simulink library "SignalSourceBlockLibrary"  (R2022b)
settings: Solver=VariableStepAuto  StartTime=0.0  StopTime=10.0  RelTol=1e-3
settings Model: Creator=isaacito  LastModifiedBy=isaacito

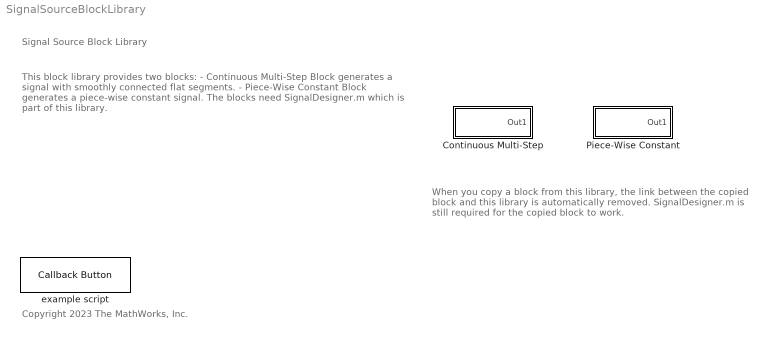
== system SignalSourceBlockLibrary ==
  note: When you copy a block from this library,
      | the link between the copied block and
      | this library is automatically removed.
      | SignalDesigner.m is still required for
      | the copied block to work.
  note: Copyright 2023 The MathWorks, Inc.
  note: Signal Source Block Library
  note: This block library provides two blocks:
      |
      | - Continuous Multi-Step Block generates
      | a signal with smoothly connected flat segments.
      |
      | - Piece-Wise Constant Block generates
      | a piece-wise constant signal.
      |
      | The blocks need SignalDesigner.m which is
      | part of this library.
  Continuous Multi-Step : Subsystem  mask(Continuous Multi-Step Signal){dataPoints=[0 1 0; 3 nan 9; 6 8 7], deltaT=0.05}
      mask prompts: dataPoints "Data points"; deltaT "Interpolation step [s]"
      mask help:
      | This block generates a signal consisting of smoothly connected flat segments. Data points parameter takes an N-by-3 matrix where each row specifies a flat segment. First column and second column define start and end time of the segment, respectively. Third column defines the value of the segment. Second column can also be NaN to define a point value. Flat segments and point values are smoothly interpolated by Akima spline with the specified interpolation step.
      |
      | For example, a matrix [0 1 5; 3 nan 9; 6 8 7] for Data points defines a signal as follows. First row defines a flat segment from t=0 to t=1 of value 5. Second row defines a point at t=3 of value 9. Third row defines a flat segment from t=6 to t=8 of value 7.
      mask init:
      | sig = SignalDesigner("continuous");
      | 
      | % Initialization function can access parameter names directly
      | sig.XYData = dataPoints;
      | sig.DeltaX = deltaT;
      | 
      | update(sig)
      | 
      | xStr = "[" + num2str(sig.Data.X') + "]";
      | yStr = "[" + num2str(sig.Data.Y') + "]";
      | 
      | set_param([gcb '/1-D Lookup Table'], 'Table', yStr)
      | set_param([gcb '/1-D Lookup Table'], 'BreakpointsForDimension1', xStr)
      settings: CopyFcn=|
      | set_param(gcb,'LinkStatus','none');
      | set_param(gcb,'CopyFcn','');
      mask DialogControl PlotButton Prompt: Plot
      mask DialogControl PlotButton Callback:
      | dataPoints = eval(get_param(gcb, "dataPoints"));
      | deltaT = eval(get_param(gcb, "deltaT"));
      | 
      | sig = SignalDesigner("continuous");
      | sig.DeltaX = deltaT;
      | sig.XYData = dataPoints;
      | sig.XVarName = "Time (s)";
      | sig.YVarName = "Data";
      | update(sig)
      | plotDataPoints(sig);
      mask DialogControl Control3 Prompt: horizontal spacer 1
      mask DialogControl Control4 Prompt: horizontal spacer 2
      mask DialogControl Control5 Prompt: horizontal spacer 3
      mask Display: disp("Continuous" + newline + "Multi-Step")
  Piece-Wise Constant : Subsystem  mask(Piece-Wise Constant Signal){dataPoints=[0 1; 2 3; 4 2; 5 2]}
      mask prompts: dataPoints "Data points"
      mask help:
      | This block generates a piece-wise constant signal. Data points parameter takes an N-by-2 matrix where each row specifies a constant segment. First column defines the start time of constant segment, and second column specifies the value of it. The value continues until the value of the next segment is defined. The values of the two consecutive rows are connected with a discrete jump.
      |
      | For example, a matrix [0 6; 1 7;2 5] for Data points defines a signal as follows. First row defines a constant segment from t=0 of value 6. Second row defines a point at t=1 of value 7. Third row defines a constant segment from t=2 of value 5. The value makes a discrete jump from one segment to the next.
      mask init:
      | sig = SignalDesigner("step");
      | 
      | % Initialization function can access parameter names directly
      | sig.XYData = dataPoints;
      | 
      | update(sig)
      | 
      | xStr = "[" + num2str(sig.Data.X') + "]";
      | yStr = "[" + num2str(sig.Data.Y') + "]";
      | 
      | set_param([gcb '/1-D Lookup Table'], 'Table', yStr)
      | set_param([gcb '/1-D Lookup Table'], 'BreakpointsForDimension1', xStr)
      settings: CopyFcn=|
      | set_param(gcb,'LinkStatus','none');
      | set_param(gcb,'CopyFcn','');
      mask DialogControl PlotButton Prompt: Plot
      mask DialogControl PlotButton Callback:
      | dataPoints = eval(get_param(gcb, "dataPoints"));
      | 
      | sig = SignalDesigner("step");
      | sig.XYData = dataPoints;
      | sig.XVarName = "Time (s)";
      | sig.YVarName = "Data";
      | update(sig)
      | plotDataPoints(sig);
      mask DialogControl Control3 Prompt: invisible horizontal spacer 1
      mask DialogControl Control4 Prompt: invisible horizontal spacer 2
      mask DialogControl Control5 Prompt: invisible horizontal spacer 3
      mask Display: disp("Piece-Wise" + newline + "Constant")
  example script : CallbackButton  ButtonText=Open
      settings: ClickFcn=edit SignalDesigner_example

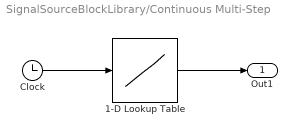
== system SignalSourceBlockLibrary/Continuous Multi-Step ==
  1-D Lookup Table : Lookup_n-D  NumberOfTableDimensions=1  BreakpointsForDimension1="[0           1        1.05         1.1        1.15         1.2        1.25         1.3        1.35         1.4        1.45         1.5        1.55         1.6        1.65         1.7        1.75         1.8        1.85         1.9        1.95           2        2.05         2.1        2.15         2.2        2.25         2.3        2.35         2.4        2.45         2.5        2.55         2.6        2.65         2.7        2.75         2.8        2.85         2.9        2.95           3        3.05         3.1        3.15         3.2        3.25         3.3        3.35         3.4        3.45         3.5        3.55         3.6        3.65         3.7        3.75         3.8        3.85         3.9        3.95           4        4.05         4.1        4.15         4.2        4.25         4.3        4.35         4.4        4.45         4.5        4.55         4.6        4.65         4.7        4.75         4.8        4.85         4.9        4.95           5        5.05         5.1        5.15         5.2        5.25         5.3        5.35         5.4        5.45         5.5        5.55         5.6        5.65         5.7        5.75         5.8        5.85         5.9        5.95           6           8]"  Table="[0           0    0.016594     0.06525     0.14428       0.252     0.38672     0.54675     0.73041       0.936      1.1618      1.4062      1.6675       1.944       2.234      2.5358      2.8477       3.168      3.4951      3.8273      4.1628         4.5      4.8372      5.1728      5.5049       5.832      6.1523      6.4643       6.766       7.056      7.3325      7.5938      7.8382       8.064      8.2696      8.4533      8.6133       8.748      8.8557      8.9348      8.9834           9      8.9984      8.9935      8.9855      8.9745      8.9606       8.944      8.9247      8.9028      8.8785      8.8519       8.823       8.792       8.759      8.7241      8.6875      8.6492      8.6093       8.568      8.5254      8.4815      8.4365      8.3905      8.3436       8.296      8.2477      8.1988      8.1495      8.0999        8.05           8        7.95      7.9001      7.8505      7.8012      7.7523       7.704      7.6564      7.6095      7.5635      7.5185      7.4746       7.432      7.3907      7.3508      7.3125      7.2759       7.241       7.208       7.177      7.1481      7.1215      7.0972      7.0753       7.056      7.0394      7.0255      7.0145      7.0065      7.0016           7           7]"  InternalRulePriority=Speed  RndMeth=Simplest
  Clock : Clock
  Out1 : Outport
  wires:
  1-D Lookup Table/1 -> Out1/1
  Clock/1 -> 1-D Lookup Table/1

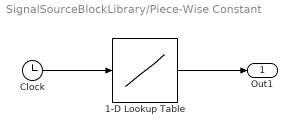
== system SignalSourceBlockLibrary/Piece-Wise Constant ==
  1-D Lookup Table : Lookup_n-D  NumberOfTableDimensions=1  BreakpointsForDimension1="[0  2  4  5]"  Table="[1  3  2  2]"  InterpMethod=Flat  InternalRulePriority=Speed  RndMeth=Simplest
  Clock : Clock
  Out1 : Outport
  wires:
  1-D Lookup Table/1 -> Out1/1
  Clock/1 -> 1-D Lookup Table/1
